simulink model "iterative_motion_controller"  (R2025a)
settings: Solver=FixedStepDiscrete  StartTime=0.0  StopTime=1  RelTol=1e-3
undefined symbols (not defined in the file): AmcfocInitConf, MAX_EVENTS_PER_TICK, N_MOTORS, Ts_ControlFOC
settings Model: DataDictionary=amcfoc.sldd  Creator=mfussi  LastModifiedBy=rpumpo
settings SolverCC: ConcurrentTasks=on  AutoInsertRateTranBlk=on  InsertRTBMode=Never (minimum delay)
settings DataIOCC: SaveOutput=off  SignalLogging=off  DSMLogging=off  SaveTime=off
settings OptimizationCC: DefaultParameterBehavior=Inlined  GainParamInheritBuiltInType=on  UseFloatMulNetSlope=on  DefaultUnderspecifiedDataType=single  UseSpecifiedMinMax=on  InlineInvariantSignals=on  PassReuseOutputArgsAs=Individual arguments  ZeroExternalMemoryAtStartup=off  ZeroInternalMemoryAtStartup=off  SimCompilerOptimization=on  OptimizeBlockOrder=speed  DifferentSizesBufferReuse=on  EfficientTunableParamExpr=on
settings DebuggingCC: AllowSymbolicDim=off
settings HardwareCC: ProdBitPerPointer=32.0  ProdBitPerSizeT=32.0  ProdBitPerPtrDiffT=32.0  ProdLargestAtomicInteger=Long  ProdLargestAtomicFloat=Double  ProdWordSize=32.0  ProdHWDeviceType=ARM Compatible->ARM Cortex-M
settings ModelReferenceCC: UpdateModelReferenceTargets=IfOutOfDate  EnableRefExpFcnMdlSchedulingChecks=on  EnableParallelModelReferenceBuilds=on  ModelReferenceNumInstancesAllowed=Single
settings SFSimCC: MATLABDynamicMemAlloc=off
settings RTWCC: SystemTargetFile=ert.tlc  GenCodeOnly=on  PackageGeneratedCodeAndArtifacts=on  TemplateMakefile=ert_default_tmf  GenerateReport=on  RTWUseSimCustomCode=on  BuildConfiguration=Faster Runs  LaunchReport=on  TargetLang=C++  GenerateCodeMetricsReport=on  GenerateCodeReplacementReport=on  GPUComputeCapability=3.5  Description=Embedded Coder
settings CodeAppCC: ForceParamTrailComments=on  IgnoreCustomStorageClasses=off  MaxIdLength=60.0  OperatorAnnotations=on  SimulinkDataObjDesc=on  SFDataObjDesc=on  InsertBlockDesc=on
settings ERTTargetCC: ExtModeTransport=0.0  ExtModeStaticAlloc=off  ExtModeMexFile=ext_comm  ExtModeIntrfLevel=Level1  RootIOFormat=Structure reference  ERTCustomFileTemplate=example_file_process.tlc  DynamicArrayContainerType=coder::array  TargetLangStandard=C++03 (ISO)  CodeReplacementLibrary=iCubTech  CombineSignalStateStructs=on  SuppressErrorStatus=on  SupportNonFinite=off

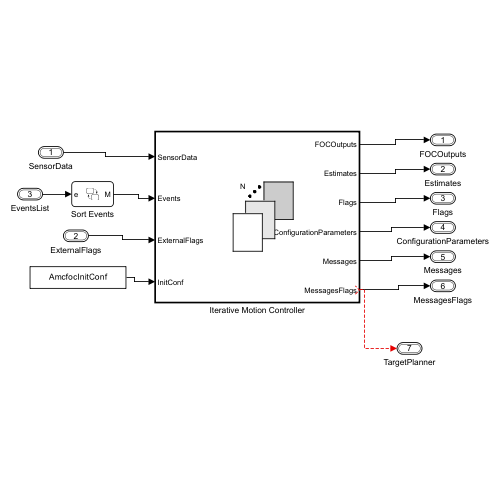
[thumbnail: Simulink's stored preview of the top-level diagram]
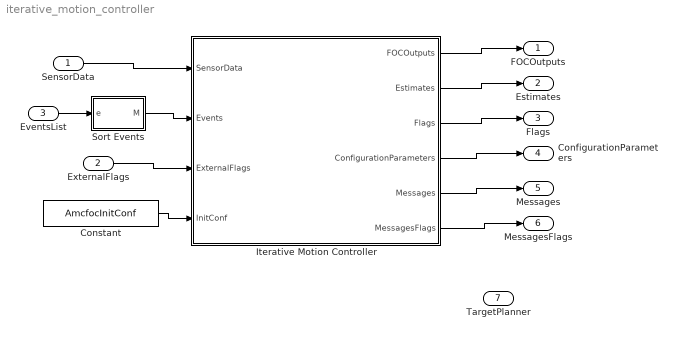
== system iterative_motion_controller ==
  SensorData : Inport  OutDataTypeStr=Bus: SensorsData  PortDimensions=N_MOTORS  SampleTime=Ts_ControlFOC  BusOutputAsStruct=on
  ExternalFlags : Inport  Port=2  OutDataTypeStr=Bus: ExternalFlags  BusOutputAsStruct=on
  EventsList : Inport  Port=3  OutDataTypeStr=Bus: ReceivedEvents  PortDimensions=N_MOTORS*MAX_EVENTS_PER_TICK  BusOutputAsStruct=on
  Constant : Constant  Value=AmcfocInitConf  OutDataTypeStr=Bus: ActuatorConfiguration  SampleTime=1e-3
  Iterative Motion Controller : Subsystem  TreatAsAtomicUnit=on
  Sort Events : Stateflow chart  TreatAsAtomicUnit=on
  FOCOutputs : Outport  OutDataTypeStr=Bus: FOCOutputs  BusOutputAsStruct=on
  Estimates : Outport  Port=2  OutDataTypeStr=Bus: EstimatedData  BusOutputAsStruct=on
  Flags : Outport  Port=3  OutDataTypeStr=Bus: Flags  BusOutputAsStruct=on
  ConfigurationParameters : Outport  Port=4  OutDataTypeStr=Bus: ActuatorConfiguration  BusOutputAsStruct=on
  Messages : Outport  Port=5  OutDataTypeStr=Bus: BUS_MESSAGES_TX  BusOutputAsStruct=on
  MessagesFlags : Outport  Port=6  OutDataTypeStr=Bus: BUS_STATUS_TX  BusOutputAsStruct=on
  TargetPlanner : Outport  Port=7  OutDataTypeStr=Bus: Targets  BusOutputAsStruct=on
  wires:
  SensorData/1 -> Iterative Motion Controller/1(SensorData)
  Iterative Motion Controller/1(FOCOutputs) -> FOCOutputs/1
  Iterative Motion Controller/2(Estimates) -> Estimates/1
  ExternalFlags/1 -> Iterative Motion Controller/3(ExternalFlags)
  Constant/1 -> Iterative Motion Controller/4(InitConf)
  Iterative Motion Controller/3(Flags) -> Flags/1
  Iterative Motion Controller/4(ConfigurationParameters) -> ConfigurationParameters/1
  EventsList/1 -> Sort Events/1(e)
  Iterative Motion Controller/5(Messages) -> Messages/1
  Iterative Motion Controller/6(MessagesFlags) -> MessagesFlags/1
  Sort Events/1(M) -> Iterative Motion Controller/2(Events)
  ? -> TargetPlanner/1

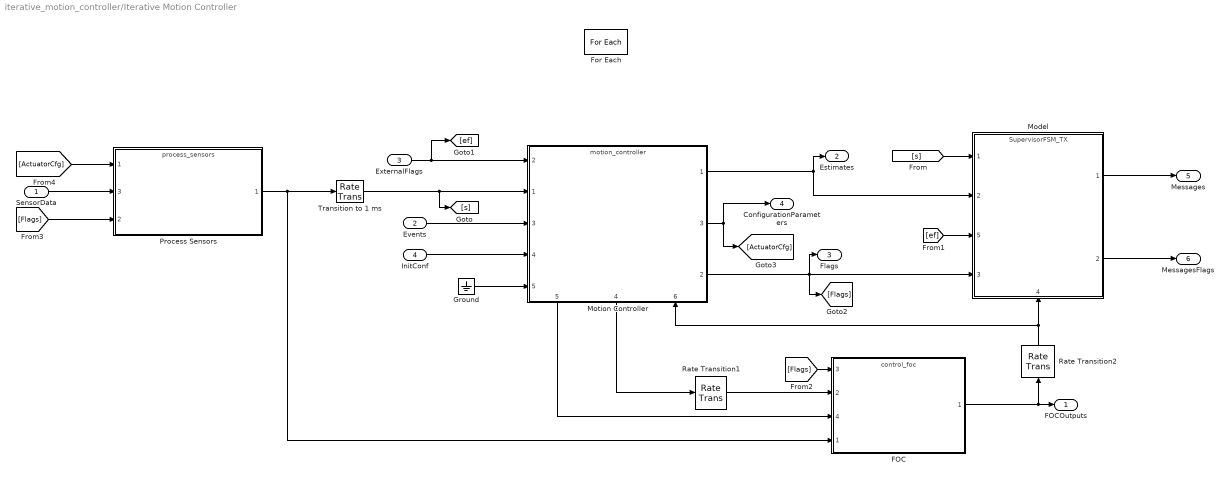
== system iterative_motion_controller/Iterative Motion Controller ==
  SensorData : Inport  OutDataTypeStr=Bus: SensorsData  Partition=on  PartitionDimension=1  PartitionWidth=1  PartitionOffset=0
  Events : Inport  Port=2  OutDataTypeStr=Bus:ReceivedEvents  Partition=on  PartitionDimension=1  PartitionWidth=1  PartitionOffset=0
  ExternalFlags : Inport  Port=3  OutDataTypeStr=Bus: ExternalFlags
  InitConf : Inport  Port=4  OutDataTypeStr=Bus: ActuatorConfiguration  Partition=on  PartitionDimension=1  PartitionWidth=1  PartitionOffset=0
  FOC : ModelReference  ModelNameDialog=control_foc.slx  ModelReferenceVersion=9.15
      settings: PortSchema="{\"entries\":[{\"content\":{\"sides\":[{\"content\":{\"connectorIds\":[\"In3\",\"In2\",\"In4\",\"In1\"]},\"type\":\"ConnectorPlacement.EquallySpacedRectSide\",\"uuid\":\"64035845-0c3f-464a-a472-f552ce65cf51\"},{\"content\":{\"connectorIds\":[\"Out1\"],\"side\":\"RIGHT\"},\"type\":\"ConnectorPlacement.EquallySpacedRectSide\",\"uuid\":\"d77f6ed4-b4df-430e-b619-ad17cd6a1f84\"},{\"content\":{\"side\":\"TOP\"},\"type\":\"ConnectorPlacement.EquallySpacedRectSide\",\"uuid\":\"9af7b88b-046d-4886-a157-b74478c37db6\"}]},\"type\":\"ConnectorPlacement.EquallySpacedConnector\",\"uuid\":\"3690b9dd-ed6b-4145-a2ff-d98778ed67fe\"}],\"packageUris\":[\"http://schema.mathworks.com/mf0/Connector/R2020b\"],\"version\":\"1.0\"}"
  For Each : ForEach  DisableCoverage=on
  Ground : Ground
  Model : ModelReference  ModelNameDialog=SupervisorFSM_TX.slx  ModelReferenceVersion=10.23
      settings: PortSchema="{\"entries\":[{\"content\":{\"sides\":[{\"content\":{\"connectorIds\":[\"In1\",\"In2\",\"In5\",\"In3\"]},\"type\":\"ConnectorPlacement.EquallySpacedRectSide\",\"uuid\":\"da3a0c31-d41a-44f2-85ec-d1033079ee97\"},{\"content\":{\"connectorIds\":[\"Out1\",\"Out2\"],\"side\":\"RIGHT\"},\"type\":\"ConnectorPlacement.EquallySpacedRectSide\",\"uuid\":\"20109ca7-306f-4d99-aef0-3fab938882d1\"},{\"content\":{\"side\":\"TOP\"},\"type\":\"ConnectorPlacement.EquallySpacedRectSide\",\"uuid\":\"7be952f9-d28b-4eac-8fc6-f95f374eaa80\"},{\"content\":{\"connectorIds\":[\"In4\"],\"side\":\"BOTTOM\"},\"type\":\"ConnectorPlacement.EquallySpacedRectSide\",\"uuid\":\"4258288d-da37-4e3f-a5e7-f71f9227c286\"}]},\"type\":\"ConnectorPlacement.EquallySpacedConnector\",\"uuid\":\"a950c446-ce16-41c8-9269-d83d512a5505\"}],\"packageUris\":[\"http://schema.mathworks.com/mf0/Connector/R2020b\"],\"version\":\"1.0\"}"
  Motion Controller : ModelReference  ModelNameDialog=motion_controller.slx  ModelReferenceVersion=5.66
      settings: PortSchema="{\"entries\":[{\"content\":{\"sides\":[{\"content\":{\"connectorIds\":[\"In2\",\"In1\",\"In3\",\"In4\",\"In5\"]},\"type\":\"ConnectorPlacement.EquallySpacedRectSide\",\"uuid\":\"379a1b60-57a2-4ccb-a061-d06c9ad096ee\"},{\"content\":{\"connectorIds\":[\"Out1\",\"Out3\",\"Out2\"],\"side\":\"RIGHT\"},\"type\":\"ConnectorPlacement.EquallySpacedRectSide\",\"uuid\":\"27b3d028-7796-406c-a973-a0b783b604b2\"},{\"content\":{\"side\":\"TOP\"},\"type\":\"ConnectorPlacement.EquallySpacedRectSide\",\"uuid\":\"38e048f9-e5c6-4a39-8bca-9fbf31731ae5\"},{\"content\":{\"connectorIds\":[\"Out5\",\"Out4\",\"In6\"],\"side\":\"BOTTOM\"},\"type\":\"ConnectorPlacement.EquallySpacedRectSide\",\"uuid\":\"75bb32c7-946e-48bf-8b37-adef3216d3a5\"}]},\"type\":\"ConnectorPlacement.EquallySpacedConnector\",\"uuid\":\"97b4f620-742c-4215-a432-9dc15dd496c6\"}],\"packageUris\":[\"http://schema.mathworks.com/mf0/Connector/R2020b\"],\"version\":\"1.0\"}"
  Process Sensors : ModelReference  ModelNameDialog=process_sensors.slx  ModelReferenceVersion=1.13
      settings: PortSchema="{\"entries\":[{\"content\":{\"sides\":[{\"content\":{\"connectorIds\":[\"In1\",\"In3\",\"In2\"]},\"type\":\"ConnectorPlacement.EquallySpacedRectSide\",\"uuid\":\"d8164f8b-a8b8-460b-bc12-0c4317305223\"},{\"content\":{\"connectorIds\":[\"Out1\"],\"side\":\"RIGHT\"},\"type\":\"ConnectorPlacement.EquallySpacedRectSide\",\"uuid\":\"a4e8ef23-f4fb-4635-b2ec-8d21946d9f16\"},{\"content\":{\"side\":\"TOP\"},\"type\":\"ConnectorPlacement.EquallySpacedRectSide\",\"uuid\":\"5aa839e4-3c8b-4cff-a1be-1b7cc5f65bac\"}]},\"type\":\"ConnectorPlacement.EquallySpacedConnector\",\"uuid\":\"a9fb15ab-116a-44d0-b290-f7a739ffe6a3\"}],\"packageUris\":[\"http://schema.mathworks.com/mf0/Connector/R2020b\"],\"version\":\"1.0\"}"
  Rate Transition1 : RateTransition  Deterministic=off  OutPortSampleTime=Ts_ControlFOC
  Rate Transition2 : RateTransition  Deterministic=off  OutPortSampleTime=Ts_Supervision
  Transition to 1 ms : RateTransition  Deterministic=off  OutPortSampleTime=Ts_Supervision
  FOCOutputs : Outport  OutDataTypeStr=Bus: FOCOutputs  ConcatenationDimension=1
  Estimates : Outport  Port=2  OutDataTypeStr=Bus: EstimatedData  ConcatenationDimension=1
  Flags : Outport  Port=3  OutDataTypeStr=Bus: Flags  ConcatenationDimension=1
  ConfigurationParameters : Outport  Port=4  OutDataTypeStr=Bus: ActuatorConfiguration  ConcatenationDimension=1
  Messages : Outport  Port=5  ConcatenationDimension=1
  MessagesFlags : Outport  Port=6  ConcatenationDimension=1
  wires:
  ExternalFlags/1 -> [ef], Motion Controller/2
  Motion Controller/4 -> Rate Transition1/1
  InitConf/1 -> Motion Controller/4
  Events/1 -> Motion Controller/3
  [s] -> Model/1
  [ef] -> Model/5
  Model/1 -> Messages/1
  Model/2 -> MessagesFlags/1
  Ground/1 -> Motion Controller/5
  Motion Controller/1 -> Estimates/1, Model/2
  Motion Controller/3 -> ConfigurationParameters/1, [ActuatorCfg]
  Transition to 1 ms/1 -> [s], Motion Controller/1
  FOC/1 -> Rate Transition2/1, FOCOutputs/1
  Rate Transition2/1 -> Model/4, Motion Controller/6
  Motion Controller/2 -> Flags/1, [Flags], Model/3
  Rate Transition1/1 -> FOC/2
  Motion Controller/5 -> FOC/4
  Process Sensors/1 -> FOC/1, Transition to 1 ms/1
  [Flags] -> FOC/3
  [Flags] -> Process Sensors/2
  SensorData/1 -> Process Sensors/3
  [ActuatorCfg] -> Process Sensors/1

== stateflow chart iterative_motion_controller/Sort Events ==
  settings: initializeOutput=1
  (default) -> (junction 13) : % Bin Events
  (junction 13) -> (junction 15) : {idx = 0;
      | counter_motor_1 = 0;
      | counter_motor_2 = 0;}
  (junction 15) -> (junction 14) [order 1] : [idx < N_MOTORS*MAX_EVENTS_PER_TICK]
  (junction 14) -> (junction 60) [order 1] : [e[idx].motor_id == 0 && counter_motor_1 < MAX_EVENTS_PER_TICK]{
      | M[e[idx].motor_id][counter_motor_1] = e[idx];
      | counter_motor_1++;}
  (junction 14) -> (junction 61) [order 2] : [e[idx].motor_id == 1 && counter_motor_2 < MAX_EVENTS_PER_TICK]{
      | M[e[idx].motor_id][counter_motor_2 ] = e[idx];
      | counter_motor_2++;}
  (junction 17) -> (junction 15) : {idx++;}
  (junction 14) -> (junction 17) [order 3]
  (junction 60) -> (junction 61)
  (junction 15) -> (junction 59) [order 2]
  (junction 61) -> (junction 17)
  data: e input Bus: ReceivedEvents size=[N_MOTORS*MAX_EVENTS_PER_TICK]; M output Bus: ReceivedEvents size=[N_MOTORS, MAX_EVENTS_PER_TICK]; idx local uint8 size=1; counter_motor_1 local uint8 size=1; counter_motor_2 local uint8 size=1; MAX_EVENTS_PER_TICK parameter; N_MOTORS parameter
